simulink subsystem "SubsMotorEcuacionesDiferenciales"  (R2023b)
settings: Solver=VariableStepAuto  StartTime=0.0  StopTime=10.0  RelTol=1e-3
undefined symbols (not defined in the file): B, J, km, L, R, Ra
settings Model: Creator=USUARIO  LastModifiedBy=USUARIO

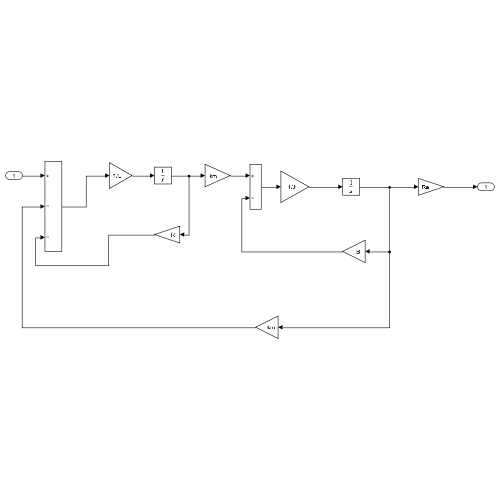
[thumbnail: Simulink's stored preview of the top-level diagram]
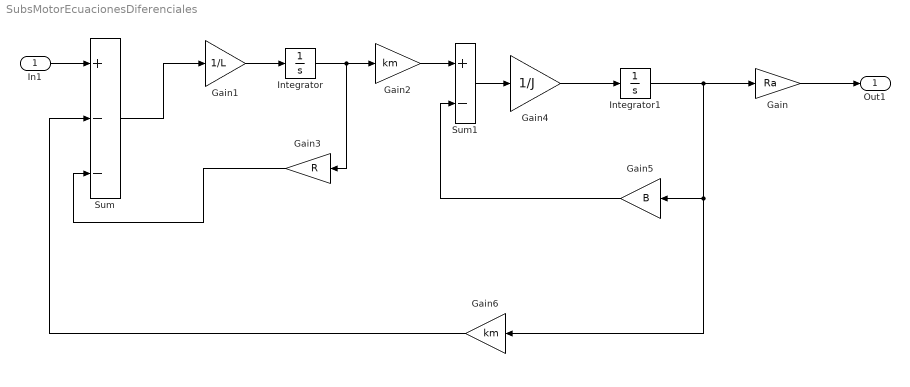
== system SubsMotorEcuacionesDiferenciales ==
  In1 : Inport
  Gain : Gain  Gain=Ra
  Gain1 : Gain  Gain=1/L
  Gain2 : Gain  Gain=km
  Gain3 : Gain  Gain=R
  Gain4 : Gain  Gain=1/J
  Gain5 : Gain  Gain=B
  Gain6 : Gain  Gain=km
  Integrator : Integrator
  Integrator1 : Integrator
  Sum : Sum  Inputs=+--
  Sum1 : Sum  Inputs=+-
  Out1 : Outport
  wires:
  Sum1/1 -> Gain4/1
  Gain5/1 -> Sum1/2
  In1/1 -> Sum/1
  Gain4/1 -> Integrator1/1
  Sum/1 -> Gain1/1
  Integrator/1 -> Gain3/1, Gain2/1
  Gain2/1 -> Sum1/1
  Gain1/1 -> Integrator/1
  Gain6/1 -> Sum/2
  Gain3/1 -> Sum/3
  Integrator1/1 -> Gain6/1, Gain5/1, Gain/1
  Gain/1 -> Out1/1
